simulink model "psbcirc2ss_psb"  (Simulink 6.0)
settings: Solver=ode23tb  SolverMode=SingleTasking  StartTime=0.0  StopTime=0.2  RelTol=1e-3  AbsTol=1e-6
libraries: powerlib2 x22
settings Model: Creator=patrice  LastModifiedBy=batserve  ExtModeTrigMode=oneshot  ExtModeArmWhenConnect=off  ExtModeAutoUpdateStatusClock=off
settings DataIOCC: LimitDataPoints=off  SignalLoggingName=sigsOut
settings OptimizationCC: BlockReduction=off  BooleanDataType=off
settings DebuggingCC: SolverPrmCheckMsg=none
settings HardwareCC: TargetUnknown=on

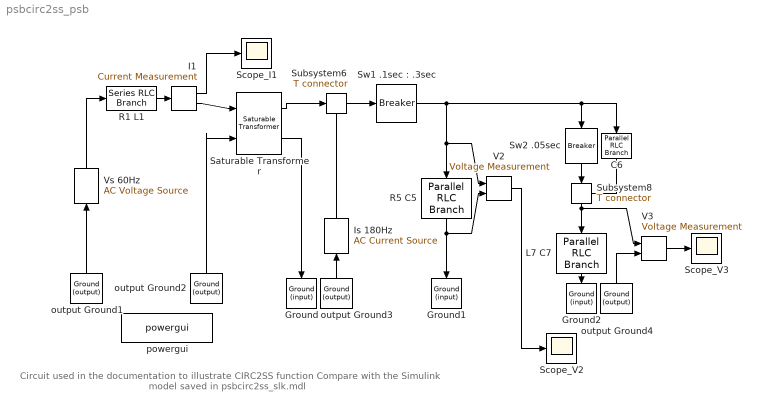
== system psbcirc2ss_psb ==
  note: Circuit used in the documentation to illustrate CIRC2SS function
      | Compare with the Simulink model saved in psbcirc2ss_slk.mdl
  C6 : powerlib2/Elements/Parallel RLC Branch  Tag=PoWeRsYsTeMbLoCk  Orientation=down  a=inf  b=inf  c=1e-09  mesure=None  PSBOutputType=1
  Ground : powerlib2/Connectors/Ground (input)  Tag=PoWeRsYsTeMbLoCk  Orientation=down
  Ground1 : powerlib2/Connectors/Ground (input)  Tag=PoWeRsYsTeMbLoCk  Orientation=down
  Ground2 : powerlib2/Connectors/Ground (input)  Tag=PoWeRsYsTeMbLoCk  Orientation=down
  I1 : powerlib2/Measurements/Current Measurement  Tag=PoWeRsYsTeMmEaSuReMeNt  PhasorSimulation=off  OutputType=Magnitude  PSBOutputType=01  PSBequivalent=0
  Is 180Hz : powerlib2/Electrical Sources/AC Current Source  Tag=PoWeRsYsTeMbLoCk  Orientation=up  A=2  P=-30  F=180  stime=0  mesure=None  PSBOutputType=1
  L7 C7 : powerlib2/Elements/Parallel RLC Branch  Tag=PoWeRsYsTeMbLoCk  Orientation=down  a=inf  b=0.5  c=2e-06  mesure=None  PSBOutputType=1
  R1 L1 : powerlib2/Elements/Series RLC Branch  Tag=PoWeRsYsTeMbLoCk  a=0.1  b=1e-03  c=inf  mesure=None  PSBOutputType=1
  R5 C5 : powerlib2/Elements/Parallel RLC Branch  Tag=PoWeRsYsTeMbLoCk  Orientation=down  a=200  b=inf  c=1e-06  mesure=None  PSBOutputType=1
  Saturable Transformer : powerlib2/Elements/Saturable Transformer  Tag=PoWeRsYsTeMbLoCk  a=[10000 60]  b=[100 0.05 1.5e-3*377]  c=[200 0.05 0]  w3check=off  d=[200 0.05 0]  e=[0 0 ; 0.001 1.2 ; 1 1.3]  f=[1000]  H=off  matfile='hysteresis'  Initialslope=+1  mesure=None  PSBOutputType=1111
  Scope_I1 : Scope
      settings: TickLabels=on  TimeRange=0.2  YMin=-15  YMax=10  DataFormat=Array
  Scope_V2 : Scope
      settings: TickLabels=on  YMin=-200  YMax=200  DataFormat=Array
  Scope_V3 : Scope
      settings: TickLabels=on  TimeRange=0.2  YMin=-400  YMax=400  DataFormat=Array
  Subsystem6 : powerlib2/Connectors/T connector  Tag=PoWeRsYsTeMbLoCk  PSBOutputType=1
  Subsystem8 : powerlib2/Connectors/T connector  Tag=PoWeRsYsTeMbLoCk  Orientation=down  PSBOutputType=1
  "Sw1 .1sec : .3sec" : powerlib2/Elements/Breaker  Tag=PoWeRsYsTeMbLoCk  a=0.01  c=1  rs=inf  cs=0  times="[ .1  .13 ]"  Ts=0  comext=off  mesure=None  PSBOutputType=1
  Sw2 .05sec : powerlib2/Elements/Breaker  Tag=PoWeRsYsTeMbLoCk  Orientation=down  a=0.1  c=0  rs=inf  cs=0  times=[ .05 ]  Ts=0  comext=off  mesure=None  PSBOutputType=1
  V2 : powerlib2/Measurements/Voltage Measurement  Tag=PoWeRsYsTeMmEaSuReMeNt  PhasorSimulation=off  OutputType=Magnitude  PSBOutputType=0  PSBequivalent=0
  V3 : powerlib2/Measurements/Voltage Measurement  Tag=PoWeRsYsTeMmEaSuReMeNt  PhasorSimulation=off  OutputType=Magnitude  PSBOutputType=0  PSBequivalent=1
  Vs 60Hz : powerlib2/Electrical Sources/AC Voltage Source  Tag=PoWeRsYsTeMbLoCk  Orientation=up  A=100  P=0  F=60  stime=0  mesure=None  PSBOutputType=1
  output Ground{1..4} (4 alike) : powerlib2/Connectors/Ground (output)  Tag=PoWeRsYsTeMbLoCk  Orientation=up  PSBOutputType=1
  powergui : powerlib2/powergui  Frange=logspace(0,3,50)  Ylog=off  Xlog=off  save=off  variable=ZData  ZoomFFT=on  StartTime=0.0  cycles=1  DisplayStyle=off  fundamental=60  FreqAxis=off  MaxFrequency=1000  frequencyindice=1  frequencyindicesteady=1  RmsSteady=1  display=off  Ts=0  methode=off  frequency=60  echomessages=off
  wires:
  Vs 60Hz/1 -> R1 L1/1
  output Ground1/1 -> Vs 60Hz/1
  Saturable Transformer/2 -> Ground/1
  output Ground2/1 -> Saturable Transformer/2
  Saturable Transformer/1 -> Subsystem6/1
  Subsystem6/1 -> "Sw1 .1sec : .3sec"/1
  R1 L1/1 -> I1/1
  I1/2 -> Saturable Transformer/1
  Sw2 .05sec/1 -> Subsystem8/1
  L7 C7/1 -> Ground2/1
  C6/1 -> Subsystem8/Enable
  Subsystem8/1 -> L7 C7/1, V3/1
  output Ground4/1 -> V3/2
  I1/1 -> Scope_I1/1
  V3/1 -> Scope_V3/1
  R5 C5/1 -> Ground1/1, V2/2
  "Sw1 .1sec : .3sec"/1 -> R5 C5/1, V2/1, Sw2 .05sec/1, C6/1
  Is 180Hz/1 -> Subsystem6/Enable
  output Ground3/1 -> Is 180Hz/1
  V2/1 -> Scope_V2/1
